simulink model "wModel_C510_BusinesJetw"  (R2020b)
settings: Solver=ode4  StartTime=0.0  StopTime=Tsim  FixedStep=0.005  RelTol=1e-3
values from neighbouring files (symbols this model uses):
  EnginePosition_Left = [-2.2; -1.26; -1.18*0]    [Model_Init00.m]
  EnginePosition_Right = [-2.2;  1.26; -1.18*0]    [Model_Init00.m]
  lat0 = 52.8259    [Model_Init00.m]
  lon0 = -1.3308    [Model_Init00.m]
  MAC = 1.57    [Model_Init00.m]
  MassKg = 3000    [Model_Init00.m]
  WingArea = 19.50    (= 19.5)    [Model_Init00.m]
  WingSpan = 13.20    (= 13.2)    [Model_Init00.m]
undefined symbols (not defined in the file or in its folder): Dx_cg, Earth, trim, WGS84
libraries: aerolibasang x3, aerolibfltsims x2, shared6dof x1, aerolibtransform2 x1, aerolibatmos2 x1
settings Model: Creator=nabram00  LastModifiedBy=kknos
settings DebuggingCC: ArithmeticOperatorsInVariantConditions=warning
settings SFSimCC: CustomCodeUndefinedFunction=UseInterfaceOnly

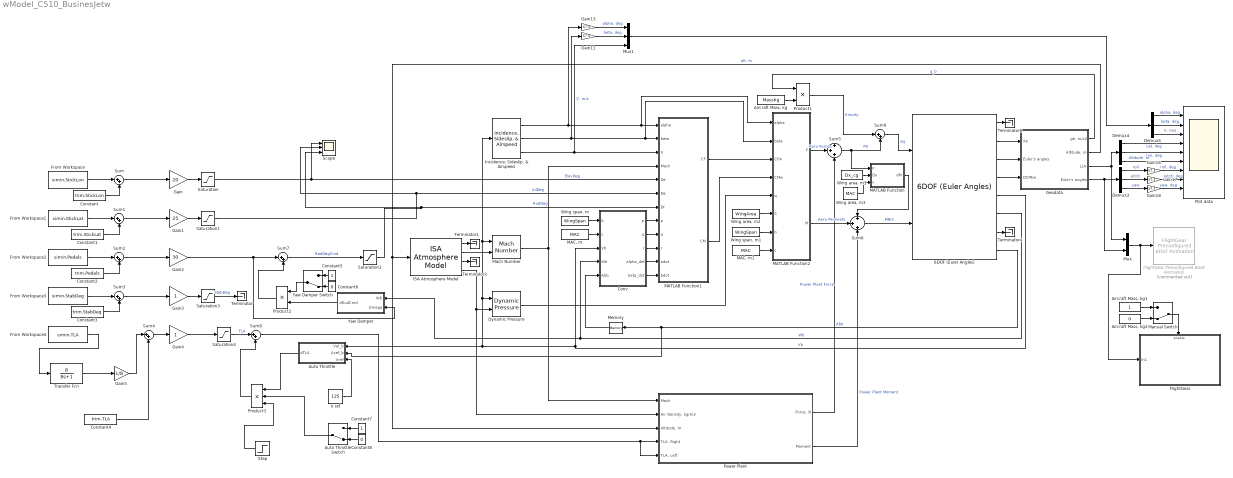
== system wModel_C510_BusinesJetw ==
  " Yaw Damper Switch" : ManualSwitch  CurrentSetting=0
  6DOF (Euler Angles) : shared6dof/6DOF (Euler Angles)  units=Metric (MKS)  mtype=Fixed  rep=Euler Angles  xme_0=trim.PositionE  Vm_0=trim.Vb  eul_0=trim.AttitudeBE  pm_0=trim.OmegaB  mass_0=MassKg  mass_e=0.5  mass_f=2.0  inertia=MoIKgM2  inertia_e=eye(3)  inertia_f=2*eye(3)  k_quat=1.0  vre_flag=on  abi_flag=off  aMode=0  xme_statename=''  Vm_statename=''  eul_statename=''  quat_statename=''  pm_statename=''  mass_statename=''
      settings: SourceProductBaseCode=AE,PW,MT,UV,VE,VP
  "Aircraft Mass, kg" : Constant  Value=MassKg
  "Aircraft Mass, kg1" : Constant  OutDataTypeStr=boolean
  "Aircraft Mass, kg2" : Constant  Value=0  OutDataTypeStr=boolean
  Auto Throttle : Subsystem
  Auto Throttle Switch : ManualSwitch  CurrentSetting=0
  Constant : Constant  Value=trim.StickLon
  Constant1 : Constant  Value=trim.StickLat
  Constant2 : Constant  Value=trim.Pedals
  Constant3 : Constant  Value=trim.StabDeg
  Constant4 : Constant  Value=trim.TLA
  Constant5 : Constant
  Constant6 : Constant  Value=0
  Constant7 : Constant
  Constant8 : Constant  Value=0
  Conv : MATLAB Function  TreatAsAtomicUnit=on
  Demux3 : Demux  Outputs=3
  Demux4 : Demux  Outputs=3
  Demux5 : Demux  Outputs=3
  Dynamic Pressure : aerolibasang/Dynamic Pressure
  FlightGear : Subsystem  TreatAsAtomicUnit=on
  FlightGear Preconfigured 6DoF Animation : aerolibfltsims/FlightGear Preconfigured 6DoF Animation  Commented=on  xFlightGearVersion=v2018.1  DestinationIpAddress=127.0.0.1  DestinationPort=5502  SampleTime=1/25  packetVersion=24
  From Workspace : FromWorkspace  VariableName=simin.StickLon
  From Workspace1 : FromWorkspace  VariableName=simin.StickLat
  From Workspace2 : FromWorkspace  VariableName=simin.Pedals
  From Workspace3 : FromWorkspace  VariableName=simin.StabDeg
  From Workspace4 : FromWorkspace  VariableName=simin.TLA
  Gain : Gain  Gain=20
  Gain1 : Gain  Gain=25
  Gain{11,13,16..18} (5 alike) : Gain  Gain=57.3
  Gain2 : Gain  Gain=30
  Gain3 : Gain
  Gain4 : Gain
  Gain5 : Gain  Gain=1/8
  Geodata : Subsystem  TreatAsAtomicUnit=on
  ISA Atmosphere Model : aerolibatmos2/ISA Atmosphere Model  custom=off  g=9.80665  gamma=1.4  R=287.0531  L=0.0065  h_trop=11000  h_strat=20000  rho0=1.225  P0=101325  T0=288.15  h0=0
  "Incidence, Sideslip, & Airspeed" : aerolibasang/Incidence, Sideslip, & Airspeed
  "MAC, m" : Constant  Value=MAC
  "MAC, m1" : Constant  Value=MAC
  MATLAB Function : MATLAB Function  TreatAsAtomicUnit=on
  MATLAB Function1 : MATLAB Function  TreatAsAtomicUnit=on
  MATLAB Function2 : MATLAB Function  TreatAsAtomicUnit=on
  Mach Number : aerolibasang/Mach Number
      settings: SourceProductBaseCode=AE
  Manual Switch : ManualSwitch  CurrentSetting=0
  Memory : Memory
  Mux : Mux  Inputs=2
  Mux1 : Mux  Inputs=3
  Plot data : Scope  NumInputPorts=9
  Power Plant : Subsystem  TreatAsAtomicUnit=on
  Product1 : Product
  Product2 : Product
  Product3 : Product  Inputs=3
  Saturation : Saturate  UpperLimit=20  LowerLimit=-20
  Saturation1 : Saturate  UpperLimit=25  LowerLimit=-25
  Saturation2 : Saturate  UpperLimit=30  LowerLimit=-30
  Saturation3 : Saturate  UpperLimit=3  LowerLimit=-8
  Saturation4 : Saturate  UpperLimit=1  LowerLimit=0
  Scope : Scope  NumInputPorts=3
  Step : Step  Time=0.1  SampleTime=0
  Sum{,1..4,7..9} (8 alike) : Sum  Inputs=|++
  Sum5 : Sum  Inputs=+|+|+
  Sum6 : Sum  Inputs=+|+|+
  Terminator{,1,3..4,6} (5 alike) : Terminator
  Transfer Fcn : TransferFcn  Numerator=[8]  Denominator=[8 1]
  V ref : Constant  Value=125
  "Wing area, m1" : Constant  Value=Dx_cg
  "Wing area, m2" : Constant  Value=WingArea
  "Wing area, m3" : Constant  Value=MAC
  "Wing span, m" : Constant  Value=WingSpan
  "Wing span, m1" : Constant  Value=WingSpan
  Yaw Damper : Subsystem
  wires:
  From Workspace/1 -> Sum/1
  From Workspace1/1 -> Sum1/1
  From Workspace2/1 -> Sum2/1
  From Workspace3/1 -> Sum3/1
  Constant/1 -> Sum/2
  Constant1/1 -> Sum1/2
  Constant2/1 -> Sum2/2
  Constant3/1 -> Sum3/2
  Constant4/1 -> Sum4/2
  Sum/1 -> Gain/1
  Sum1/1 -> Gain1/1
  Sum2/1 -> Gain2/1
  Sum3/1 -> Gain3/1
  Sum4/1 -> Gain4/1
  Gain/1 -> Saturation/1
  Gain1/1 -> Saturation1/1
  Gain3/1 -> Saturation3/1
  Gain4/1 -> Saturation4/1
  Saturation/1 -> MATLAB Function1/5(De), Scope/1  "ElevDeg"
  Saturation1/1 -> Scope/2, MATLAB Function1/6(Da)  "AilDeg"
  Saturation2/1 -> Scope/3, MATLAB Function1/7(Dr)  "RudDeg"
  Saturation3/1 -> Terminator/1  "StabDeg"
  ISA Atmosphere Model/4 -> Power Plant/2("Air Density, kg/m3"), Dynamic Pressure/2
  ISA Atmosphere Model/3 -> Terminator3/1
  ISA Atmosphere Model/2 -> Mach Number/2
  ISA Atmosphere Model/1 -> Terminator1/1
  Geodata/2("Altitude, m") -> ISA Atmosphere Model/1, Power Plant/3("Altitude, m")  "alt, m"
  MATLAB Function1/1(CF) -> MATLAB Function2/3(CFw)
  MATLAB Function1/2(CM) -> MATLAB Function2/4(CMw)
  Sum6/1 -> 6DOF (Euler Angles)/2  "MNm"
  6DOF (Euler Angles)/6 -> Conv/4(Wb), Yaw Damper/1(Wb)  "Wb"
  Conv/1(p) -> MATLAB Function1/8(p)
  Conv/2(q) -> MATLAB Function1/9(q)
  Conv/3(r) -> MATLAB Function1/10(r)
  Mach Number/1 -> MATLAB Function1/4(Mach), Power Plant/1(Mach)
  Dynamic Pressure/1 -> MATLAB Function2/5(q)
  6DOF (Euler Angles)/5 -> Auto Throttle/1(Vel_b), Mach Number/1, "Incidence, Sideslip, & Airspeed"/1, Dynamic Pressure/1, Conv/3(Vb)  "Vb"
  "Incidence, Sideslip, & Airspeed"/1 -> MATLAB Function1/1(alpha), MATLAB Function2/1(alpha), Gain13/1
  "Incidence, Sideslip, & Airspeed"/2 -> MATLAB Function1/2(beta), MATLAB Function2/2(beta), Gain11/1
  "Incidence, Sideslip, & Airspeed"/3 -> Mux1/3, MATLAB Function1/3(V)  "V, m/s"
  Mux/1 -> FlightGear/1(In1), FlightGear Preconfigured 6DoF Animation/1
  Conv/4(alpha_dot) -> MATLAB Function1/11(adot)
  Conv/5(beta_dot) -> MATLAB Function1/12(bdot)
  "Wing span, m1"/1 -> MATLAB Function2/7(b)
  "MAC, m1"/1 -> MATLAB Function2/8(c)
  Gain13/1 -> Mux1/1  "alpha, deg"
  MATLAB Function2/2(M) -> Sum6/2  "Aero Moments"
  MATLAB Function2/1(F) -> Sum5/2  "Aero Forces"
  6DOF (Euler Angles)/8 -> Auto Throttle/2(Acef_b), Memory/1  "Abb"
  6DOF (Euler Angles)/7 -> Terminator4/1
  6DOF (Euler Angles)/1 -> Terminator6/1
  6DOF (Euler Angles)/3 -> Geodata/2(Euler's angles)
  "Aircraft Mass, kg"/1 -> Product1/2
  Product1/1 -> Sum9/1  "Gravity"
  Demux3/1 -> Gain16/1  "roll"
  Demux3/2 -> Gain17/1  "pitch"
  Demux3/3 -> Gain18/1  "yaw"
  Gain16/1 -> Plot data/7  "roll, deg"
  Gain17/1 -> Plot data/8  "pitch, deg"
  Gain18/1 -> Plot data/9  "yaw, deg"
  Geodata/1("gb, m/s2") -> Product1/1  "g_b"
  6DOF (Euler Angles)/2 -> Geodata/1(Xe)
  6DOF (Euler Angles)/4 -> Geodata/3(DCMbe)
  Geodata/4(Euler's angles) -> Demux3/1, Mux/2
  Geodata/3(LLA) -> Demux4/1, Mux/1
  Demux4/1 -> Plot data/4  "Lat, deg"
  Demux4/2 -> Plot data/5  "Lon, deg"
  Demux4/3 -> Plot data/6  "Altitude, m"
  "Wing span, m"/1 -> Conv/1(b)
  "Wing area, m2"/1 -> MATLAB Function2/6(S)
  "MAC, m"/1 -> Conv/2(c)
  Power Plant/1("Force, N") -> Sum5/3  "Power Plant Force"
  Power Plant/2(Moment) -> Sum6/3  "Power Plant Moment"
  Mux1/1 -> Demux5/1
  Demux5/3 -> Plot data/3  "V, m/s"
  Demux5/2 -> Plot data/2  "beta, deg"
  Demux5/1 -> Plot data/1  "alpha, deg"
  Gain11/1 -> Mux1/2  "beta, deg"
  Manual Switch/1 -> FlightGear/Enable
  "Aircraft Mass, kg2"/1 -> Manual Switch/2
  "Aircraft Mass, kg1"/1 -> Manual Switch/1
  Memory/1 -> Conv/5(Abb)
  Gain2/1 -> Sum7/1, Yaw Damper/2(Omega)
  Sum7/1 -> Saturation2/1  "RadDegCmd"
  Yaw Damper/1(dRudCmd) -> Product2/2
  Constant5/1 -> " Yaw Damper Switch"/1
  Constant6/1 -> " Yaw Damper Switch"/2
  " Yaw Damper Switch"/1 -> Product2/1
  Product2/1 -> Sum7/2
  Constant8/1 -> Auto Throttle Switch/2
  Constant7/1 -> Auto Throttle Switch/1
  Auto Throttle/1(dTLA) -> Product3/1
  Product3/1 -> Sum8/2
  Saturation4/1 -> Sum8/1  "TLA"
  V ref/1 -> Auto Throttle/3(Vref)
  Transfer Fcn/1 -> Gain5/1
  Sum9/1 -> 6DOF (Euler Angles)/1  "FN"
  Sum5/1 -> MATLAB Function/1(F), Sum9/2  "FN"
  "Wing area, m1"/1 -> MATLAB Function/2(Dx)
  "Wing area, m3"/1 -> MATLAB Function/3(c)
  MATLAB Function/1(dM) -> Sum6/1
  From Workspace4/1 -> Transfer Fcn/1
  Auto Throttle Switch/1 -> Product3/2
  Gain5/1 -> Sum4/1
  Sum8/1 -> Power Plant/5("TLA, Left"), Power Plant/4("TLA, Right")
  Step/1 -> Product3/3

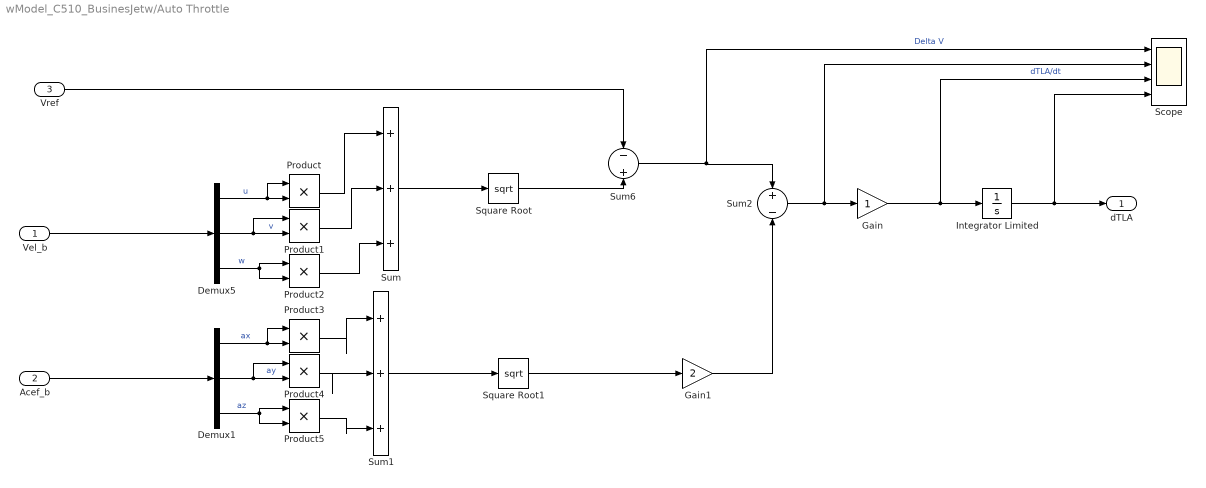
== system wModel_C510_BusinesJetw/Auto Throttle ==
  Vel_b : Inport
  Acef_b : Inport  Port=2
  Vref : Inport  Port=3
  Demux1 : Demux  Outputs=3
  Demux5 : Demux  Outputs=3
  Gain : Gain
  Gain1 : Gain  Gain=2
  Integrator Limited : Integrator  LimitOutput=on  UpperSaturationLimit=1  LowerSaturationLimit=0
  Product{,1..5} (6 alike) : Product
  Scope : Scope  NumInputPorts=4
  Square Root : Sqrt  SaturateOnIntegerOverflow=on
  Square Root1 : Sqrt  SaturateOnIntegerOverflow=on
  Sum : Sum  Inputs=|+++
  Sum1 : Sum  Inputs=|+++
  Sum2 : Sum  Inputs=+|-
  Sum6 : Sum  Inputs=-|+
  dTLA : Outport
  wires:
  Demux5/3 -> Product2/1, Product2/2  "w"
  Demux5/1 -> Product/1, Product/2  "u"
  Demux5/2 -> Product1/1, Product1/2  "v"
  Demux1/1 -> Product3/1, Product3/2  "ax"
  Demux1/3 -> Product5/1, Product5/2  "az"
  Demux1/2 -> Product4/1, Product4/2  "ay"
  Product1/1 -> Sum/2
  Product/1 -> Sum/1
  Product2/1 -> Sum/3
  Product3/1 -> Sum1/1
  Product4/1 -> Sum1/2
  Product5/1 -> Sum1/3
  Sum/1 -> Square Root/1
  Sum1/1 -> Square Root1/1
  Vref/1 -> Sum6/1
  Square Root/1 -> Sum6/2
  Sum6/1 -> Sum2/1, Scope/1  "Delta V"
  Square Root1/1 -> Gain1/1
  Gain1/1 -> Sum2/2
  Sum2/1 -> Scope/2, Gain/1
  Gain/1 -> Integrator Limited/1, Scope/3  "dTLA/dt"
  Vel_b/1 -> Demux5/1
  Acef_b/1 -> Demux1/1
  Integrator Limited/1 -> Scope/4, dTLA/1

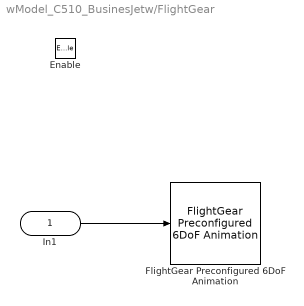
== system wModel_C510_BusinesJetw/FlightGear ==
  In1 : Inport
  Enable : EnablePort
  FlightGear Preconfigured 6DoF Animation : aerolibfltsims/FlightGear Preconfigured 6DoF Animation  xFlightGearVersion=v2018.1  DestinationIpAddress=127.0.0.1  DestinationPort=5502  SampleTime=1/25  packetVersion=24
  wires:
  In1/1 -> FlightGear Preconfigured 6DoF Animation/1

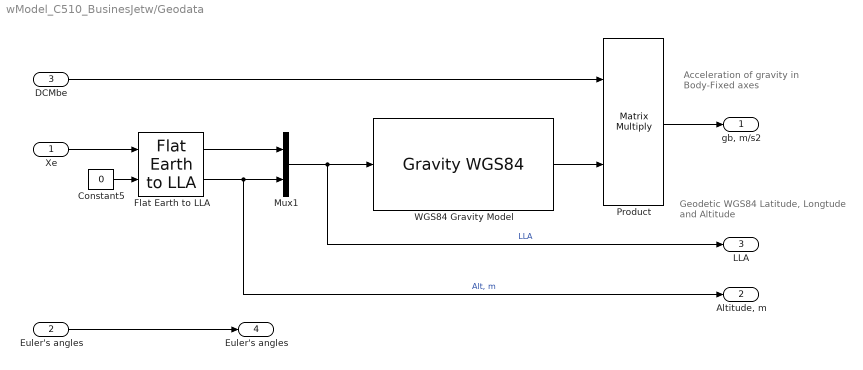
== system wModel_C510_BusinesJetw/Geodata ==
  note: Geodetic WGS84
      | Latitude, Longtude and Altitude
  note: Acceleration of gravity
      | in Body-Fixed axes
  Xe : Inport
  Euler's angles : Inport  Port=2
  DCMbe : Inport  Port=3
  Constant5 : Constant  Value=0
  Flat Earth to LLA : aerolibtransform2/Flat Earth to LLA  units=Metric (MKS)  ptype=Earth (WGS84)  F=1/298.257223563  R=6378137  refPosPort=off  LL0=[lat0 lon0]  psi=0
  Mux1 : Mux  Inputs=2
  Product : Product  Multiplication=Matrix(*)
  "WGS84 Gravity Model  " : GravityWGS84
  "gb, m/s2" : Outport  VectorParamsAs1DForOutWhenUnconnected=off
  "Altitude, m" : Outport  Port=2  VectorParamsAs1DForOutWhenUnconnected=off
  LLA : Outport  Port=3  VectorParamsAs1DForOutWhenUnconnected=off
  Euler's angles : Outport  Port=4  VectorParamsAs1DForOutWhenUnconnected=off
  wires:
  Xe/1 -> Flat Earth to LLA/1
  DCMbe/1 -> Product/1
  Product/1 -> "gb, m/s2"/1
  Flat Earth to LLA/1 -> Mux1/1
  Constant5/1 -> Flat Earth to LLA/2
  "WGS84 Gravity Model  "/1 -> Product/2
  Flat Earth to LLA/2 -> Mux1/2, "Altitude, m"/1  "Alt, m"
  Mux1/1 -> "WGS84 Gravity Model  "/1, LLA/1  "LLA"
  Euler's angles/1 -> Euler's angles/1

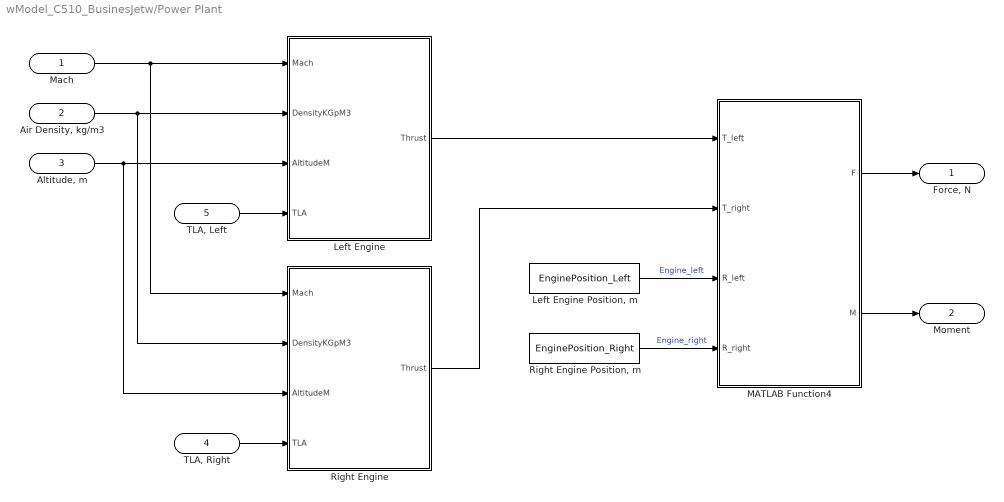
== system wModel_C510_BusinesJetw/Power Plant ==
  Mach : Inport
  "Air Density, kg/m3" : Inport  Port=2
  "Altitude, m" : Inport  Port=3
  "TLA, Right" : Inport  Port=4
  "TLA, Left" : Inport  Port=5
  Left Engine : MATLAB Function  TreatAsAtomicUnit=on
  "Left Engine Position, m" : Constant  Value=EnginePosition_Left
  MATLAB Function4 : MATLAB Function  TreatAsAtomicUnit=on
  Right Engine : MATLAB Function  TreatAsAtomicUnit=on
  "Right Engine Position, m" : Constant  Value=EnginePosition_Right
  "Force, N" : Outport  VectorParamsAs1DForOutWhenUnconnected=off
  Moment : Outport  Port=2  VectorParamsAs1DForOutWhenUnconnected=off
  wires:
  "Left Engine Position, m"/1 -> MATLAB Function4/3(R_left)  "Engine_left"
  "Right Engine Position, m"/1 -> MATLAB Function4/4(R_right)  "Engine_right"
  MATLAB Function4/1(F) -> "Force, N"/1
  Mach/1 -> Left Engine/1(Mach), Right Engine/1(Mach)
  "Air Density, kg/m3"/1 -> Left Engine/2(DensityKGpM3), Right Engine/2(DensityKGpM3)
  "Altitude, m"/1 -> Left Engine/3(AltitudeM), Right Engine/3(AltitudeM)
  "TLA, Left"/1 -> Left Engine/4(TLA)
  "TLA, Right"/1 -> Right Engine/4(TLA)
  MATLAB Function4/2(M) -> Moment/1
  Left Engine/1(Thrust) -> MATLAB Function4/1(T_left)
  Right Engine/1(Thrust) -> MATLAB Function4/2(T_right)

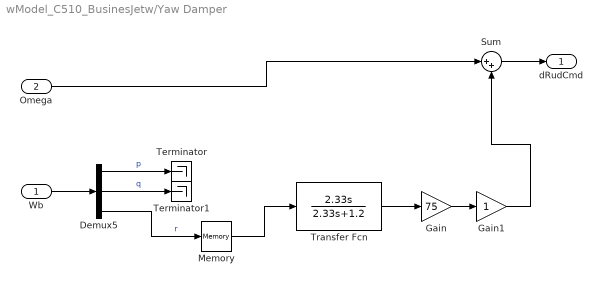
== system wModel_C510_BusinesJetw/Yaw Damper ==
  Wb : Inport
  Omega : Inport  Port=2
  Demux5 : Demux  Outputs=3
  Gain : Gain  Gain=75
  Gain1 : Gain
  Memory : Memory
  Sum : Sum  Inputs=|++
  Terminator : Terminator
  Terminator1 : Terminator
  Transfer Fcn : TransferFcn  Numerator=[2.33 0]  Denominator=[2.33 1.2]
  dRudCmd : Outport
  wires:
  Demux5/1 -> Terminator/1  "p"
  Demux5/3 -> Memory/1  "r"
  Demux5/2 -> Terminator1/1  "q"
  Wb/1 -> Demux5/1
  Transfer Fcn/1 -> Gain/1
  Gain/1 -> Gain1/1
  Gain1/1 -> Sum/2
  Omega/1 -> Sum/1
  Sum/1 -> dRudCmd/1
  Memory/1 -> Transfer Fcn/1

== matlab function wModel_C510_BusinesJetw/MATLAB Function ==
  data: F input; dM output; Dx input; c input
function dM = cg_shift(F,Dx,c)

dM = zeros(3,1);
dM = cross([-Dx*c; 0; 0],F(:));


end

== matlab function wModel_C510_BusinesJetw/MATLAB Function1 ==
  data: alpha input; beta input; V input; CF output; Mach input; De input; CM output; Da input; Dr input; p input; q input; r input; adot input; bdot input
function [CF, CM] = C510aero(alpha, beta, V, Mach, De,Da,Dr, p,q,r, adot,bdot)
%% inputs:
%  alpha, beta  - rad
%  Mach         - undim
%  De,Da,Dr     - deg
%  p,q,r        - undim
%  adot         - undim
%  bdot         - undim


AlphaTable = [-10    -8    -6    -4    -2     0     2     4     6     8    10    11    12    13    14    15    16    17    18    19    20    21    22    23    24    25    30    35    40    45    50    55    60    65    70    75    80    85    90];

%% Drag force
% Drag_at_zero_lift
CD0 = 0;

% Drag_due_to_alpha
CDTable = [ 0.0814    0.0613    0.0458    0.0347    0.0280    0.0258    0.0280    0.0347    0.0458    0.0613    0.0705    0.0811    0.0933    0.1073    0.1180    0.1298    0.1428    0.1571    0.1728    0.1901    0.2091    0.2300    0.2530    0.2783  0.3061    0.3392    0.5617    0.8479    1.1934    1.5886    2.0199    2.4698    2.9185    3.3450    3.7284    4.0495    4.2916    4.4422    4.4933];
CDwbh = interp1(AlphaTable, CDTable, rad2deg(alpha));

% Drag_due_to_Elevator_Deflection, per rad
CDDe = 0.07;

% Drag_due_to_sideslip
CDbeta = 0.16;

CD = CD0 + CDwbh + CDDe*deg2rad(De) + CDbeta*abs(beta);



%% Side force
% Side_force_due_to_beta
CYBetaTable = [-0.6489   -0.6525   -0.6553   -0.6573   -0.6585   -0.6589   -0.6585   -0.6573   -0.6553   -0.6525   -0.6489   -0.6468   -0.6445   -0.6420   -0.6393   -0.6364   -0.6334   -0.6301   -0.6266   -0.6230   -0.6191   -0.6151   -0.6109   -0.6065 -0.6019   -0.5971   -0.5706   -0.5397   -0.5047   -0.4659   -0.4235   -0.3779   -0.3294   -0.2785   -0.2254   -0.1705   -0.1144   -0.0574    0.0000];
CYb = interp1(AlphaTable, CYBetaTable, rad2deg(alpha));

% Side_force_due_to_aileron
CYda = -0.043;

% Side_force_due_to_rudder
CYdr = 0.1574;

% Side_force_due_to_roll_rate
CYp = -0.04;

% Side_force_due_to_yaw_rate
CYr = 0.233;

CY = CYb*beta + CYda*deg2rad(Da) + CYdr*deg2rad(Dr) + CYp*p + CYr*r;



%% Lift(alpha, De, adot, q)
% Lift_due_to_alpha
CLTable = [-1.1041   -0.8833   -0.6625   -0.4417   -0.2208   0    0.2208    0.4417    0.6625    0.8833    1.1041    1.2117    1.2885    1.3346    1.3500    1.3346    1.2885    1.2117    1.1041    0.9659    0.7968    0.7300    0.7300    0.7400    0.7600    0.7800    0.9728    1.2109    1.4222    1.5886    1.6949    1.7294    1.6850    1.5598    1.3570    1.0850    0.7567    0.3886   -0.0000];
CLwbh = interp1(AlphaTable, CLTable, rad2deg(alpha));

% Lift_due_to_Elevator_Deflection
CLDeTable = [0.4885    0.4912    0.4933    0.4948    0.4957    0.4956    0.4951    0.4937    0.4915    0.4882    0.4835    0.4805    0.4769    0.4727    0.4677    0.4619    0.4550    0.4468    0.4373    0.4263    0.4136    0.3994    0.3837    0.3667    0.3488    0.3306    0.2505    0.2058    0.1827    0.1660    0.1503    0.1339    0.1167    0.0987    0.0798    0.0604    0.0405    0.0203   -0.0000];
CLDe = interp1(AlphaTable, CLDeTable, rad2deg(alpha));

% Lift_due_to_alpha_rate
CLadot = 2.24;

% Lift_due_to_pitch_rate
CLq  = 4.49;

CL = CLwbh + CLDe*deg2rad(De) + CLadot*adot + CLq*q;



%% Roll
% Roll_moment_due_to_beta
ClBetaTable = [0.0027   -0.0068   -0.0164   -0.0261   -0.0358   -0.0454   -0.0550   -0.0646   -0.0740   -0.0832   -0.0922   -0.0965   -0.0995   -0.1011   -0.1013   -0.1002   -0.0978   -0.0940   -0.0891   -0.0828   -0.0754   -0.0722   -0.0717   -0.0716  -0.0718   -0.0720   -0.0761   -0.0805   -0.0824   -0.0812   -0.0768   -0.0694   -0.0595   -0.0480   -0.0358   -0.0240   -0.0136   -0.0054    0.0000];
Clb = interp1(AlphaTable, ClBetaTable, rad2deg(alpha));

% Roll_moment_due_to_roll_rate_(roll_damping)
ClpTable = [-0.7476   -0.7517   -0.7549   -0.7572   -0.7586   -0.7591   -0.7586   -0.7572   -0.7549   -0.7517   -0.7476   -0.7452   -0.7425   -0.7396   -0.7365   -0.7332   -0.7297   -0.7259   -0.7219   -0.7177   -0.7133   -0.7087   -0.7038   -0.6988    -0.6935   -0.6880   -0.6574   -0.6218   -0.5815   -0.5368   -0.4879   -0.4354   -0.3795   -0.3208   -0.2596   -0.1965   -0.1318   -0.0662    0.0000];
Clp = interp1(AlphaTable, ClpTable, rad2deg(alpha));

% Roll_moment_due_to_yaw_rate
ClrTable = [-0.7476   -0.7517   -0.7549   -0.7572   -0.7586   -0.7591   -0.7586   -0.7572   -0.7549   -0.7517   -0.7476   -0.7452   -0.7425   -0.7396   -0.7365   -0.7332   -0.7297   -0.7259   -0.7219   -0.7177   -0.7133   -0.7087   -0.7038   -0.6988    -0.6935   -0.6880   -0.6574   -0.6218   -0.5815   -0.5368   -0.4879   -0.4354   -0.3795   -0.3208   -0.2596   -0.1965   -0.1318   -0.0662    0.0000];
Clr = interp1(AlphaTable, ClrTable, rad2deg(alpha));

% Roll_moment_due_to_aileron
ClDaTable = [0.1099    0.1105    0.1110    0.1113    0.1115    0.1116    0.1115    0.1113    0.1110    0.1105    0.1099    0.1095    0.1091    0.1087    0.1083    0.1078    0.1073    0.1067    0.1061    0.1055    0.1048    0.1042    0.1035    0.1027    0.1019    0.1011    0.0966    0.0914    0.0855    0.0789    0.0717    0.0640    0.0558    0.0472    0.0382    0.0289    0.0194    0.0097   -0.0000];
Clda = interp1(AlphaTable, ClDaTable, rad2deg(alpha));

% Roll_moment_due_to_rudder
ClDrTable = [-0.0383   -0.0385   -0.0386   -0.0388   -0.0388   -0.0389   -0.0388   -0.0388   -0.0386   -0.0385   -0.0383   -0.0381   -0.0380   -0.0379   -0.0377   -0.0375   -0.0374   -0.0372   -0.0370   -0.0367   -0.0365   -0.0363   -0.0360   -0.0358    -0.0355   -0.0352   -0.0337   -0.0318   -0.0298   -0.0275   -0.0250   -0.0223   -0.0194   -0.0164   -0.0133   -0.0101   -0.0067   -0.0034    0.0000];
Cldr = interp1(AlphaTable, ClDrTable, rad2deg(alpha));

Cl = Clb*beta + Clda*deg2rad(Da) + Cldr*deg2rad(Dr) + Clp*p + Clr*r;



%% Pitch moment (alpha, q, adot, De)
% Pitching_moment_at_zero_alpha
Cmo = 0.02;

% Pitch_moment_due_to_alpha
CmTable = [0.1467    0.1176    0.0884    0.0590    0.0295         0   -0.0295   -0.0590   -0.0884   -0.1176   -0.1464   -0.1605   -0.1704   -0.1764   -0.1782   -0.1761   -0.1702   -0.1604   -0.1469   -0.1299   -0.1092   -0.0983   -0.0885   -0.0796          -0.0717   -0.0755   -0.1223   -0.1940   -0.2537   -0.3070   -0.3603   -0.4120   -0.4605   -0.5043   -0.5421   -0.5728   -0.5954   -0.6093   -0.6139];
Cmalpha = interp1(AlphaTable, CmTable, rad2deg(alpha));

% Pitch_moment_due_to_pitch_rate
Cmq = -13.17;

% Pitch_moment_due_to_alpha_rate
Cmadot = -7.42;

% Pitch_moment_due_to_elevator_deflection
CmDeTable = [-1.5323   -1.5408   -1.5474   -1.5521   -1.5549   -1.5547   -1.5530   -1.5488   -1.5417   -1.5313   -1.5166   -1.5071   -1.4960   -1.4828   -1.4672   -1.4488   -1.4271   -1.4015   -1.3717   -1.3371   -1.2975   -1.2528   -1.2034   -1.1501   -1.0941   -1.0369   -0.7858   -0.6456   -0.5731   -0.5208   -0.4714   -0.4201   -0.3661   -0.3094   -0.2504   -0.1895   -0.1271   -0.0638    0.0000];
Cmde = interp1(AlphaTable, CmDeTable, rad2deg(alpha));

Cm = Cmo + Cmalpha + Cmq*q + Cmadot*adot + Cmde*deg2rad(De);



%% Yaw moment
% Yaw_moment_due_to_beta
CnBetaTable = [0.0945    0.0959    0.0972    0.0983    0.0994    0.1003    0.1011    0.1018    0.1023    0.1028    0.1030    0.1031    0.1031    0.1028    0.1025    0.1019    0.1013    0.1005    0.0995    0.0984    0.0972    0.0963    0.0957    0.0950    0.0944    0.0937    0.0902    0.0861    0.0811    0.0753    0.0687    0.0614    0.0535    0.0450    0.0361    0.0271    0.0179    0.0089   -0.0000];
Cnb = interp1(AlphaTable, CnBetaTable, rad2deg(alpha));

% Yaw_moment_due_to_roll_rate
CnpTable = [0.1536    0.1236    0.0931    0.0623    0.0312         0   -0.0312   -0.0623   -0.0931   -0.1236   -0.1536   -0.1681   -0.1781   -0.1838   -0.1851   -0.1822   -0.1750   -0.1637   -0.1484   -0.1290   -0.1058   -0.0963   -0.0956   -0.0963   -0.0981   -0.0999   -0.1190   -0.1402   -0.1539   -0.1587   -0.1539   -0.1402   -0.1190   -0.0931   -0.0656   -0.0397   -0.0186   -0.0048   -0.0000];
Cnp = interp1(AlphaTable, CnpTable, rad2deg(alpha));

% Yaw_moment_due_to_yaw_rate
CnrTable = [-0.1883   -0.1445   -0.1102   -0.0855   -0.0706   -0.0656   -0.0706   -0.0855   -0.1102   -0.1445   -0.1883   -0.2128   -0.2314   -0.2427   -0.2458   -0.2406   -0.2274   -0.2074   -0.1818   -0.1529   -0.1231   -0.1125   -0.1117   -0.1123    -0.1143   -0.1162   -0.1412   -0.1775   -0.2098   -0.2302   -0.2324   -0.2143   -0.1790   -0.1336   -0.0873   -0.0484   -0.0216   -0.0071    0.0000];
Cnr = interp1(AlphaTable, CnrTable, rad2deg(alpha));

% Yaw_moment_due_to_aileron
CnDaTable   = [0     0     0     0     0     0     0     0     0     0     0     0     0     0     0     0     0     0     0     0     0     0     0     0     0     0     0     0     0     0     0     0     0     0     0     0     0     0     0];
Cnda = interp1(AlphaTable, CnDaTable, rad2deg(alpha));

% Yaw_moment_due_to_rudder
CnDrTable   = [-0.0917   -0.0922   -0.0926   -0.0929   -0.0931   -0.0931   -0.0931   -0.0929   -0.0926   -0.0922   -0.0917   -0.0914   -0.0911   -0.0907   -0.0904   -0.0900   -0.0895   -0.0891   -0.0886   -0.0881   -0.0875   -0.0869   -0.0863   -0.0857    -0.0851   -0.0844   -0.0807   -0.0763   -0.0713   -0.0659   -0.0599   -0.0534   -0.0466   -0.0394   -0.0319   -0.0241   -0.0162   -0.0081    0.0000];
Cndr = interp1(AlphaTable, CnDrTable, rad2deg(alpha));

Cn  = Cnb*beta + Cnp*p + Cnr*r + Cnda*deg2rad(Da) + Cndr*deg2rad(Dr);



%% In wind axes
CF = [CD CY CL]';
CM = [Cl Cm Cn]';

end

== matlab function wModel_C510_BusinesJetw/Power Plant/Left Engine ==
  data: Mach input; DensityKGpM3 input; AltitudeM input; TLA input; Thrust output
function Thrust  = BJprop(Mach,DensityKGpM3,AltitudeM,TLA)

StaticThrust = 6490;	% Static thrust at sea level, N	
Thrust       = TLA*StaticThrust*(DensityKGpM3/1.225)^0.7*(1-exp((AltitudeM-17000)/2000)); 	% Thrust at Altitude, N 

end

== matlab function wModel_C510_BusinesJetw/MATLAB Function2 ==
  data: alpha input; beta input; CFw input; F output; CMw input; q input; S input; b input; c input; M output
function [F,M] = Conv2Dim(alpha, beta, CFw, CMw, q, S, b, c)
% Computation of dimensional forces and moments

F = zeros(3,1);
M = zeros(3,1);

% Convertion from wind to body frame, ignore sideslip
CX = -CFw(1)*cos(alpha) + CFw(3)*sin(alpha);
CY =  CFw(2);
CZ = -CFw(1)*sin(alpha) - CFw(3)*cos(alpha);

% Dimensional aerodynamic forces and moments
F(1) = CX * q*S;  % N
F(2) = CY * q*S;  % N
F(3) = CZ * q*S;  % N

M(1) = CMw(1) * q*S*b;  % Nm
M(2) = CMw(2) * q*S*c;  % Nm
M(3) = CMw(3) * q*S*b;  % Nm
 
end

== matlab function wModel_C510_BusinesJetw/Power Plant/Right Engine ==
  data: Mach input; DensityKGpM3 input; AltitudeM input; TLA input; Thrust output
function Thrust  = BJprop(Mach,DensityKGpM3,AltitudeM,TLA)

StaticThrust = 6490;	% Static thrust at sea level, N	
Thrust       = TLA*StaticThrust*(DensityKGpM3/1.225)^0.7*(1-exp((AltitudeM-17000)/2000)); 	% Thrust at Altitude, N 

end

== matlab function wModel_C510_BusinesJetw/Power Plant/MATLAB Function4 ==
  data: T_left input; T_right input; R_left input; R_right input; F output; M output
function [F,M] = PowerPlantFM(T_left, T_right, R_left, R_right)

F = zeros(3,1);
M = zeros(3,1);

% Total force (Thrust axes is parallel to xb)
F(1) = T_left + T_right; % N

% Moments from left and right engine, Nm
M_left  = cross(R_left,  [T_left;  0; 0]);
M_right = cross(R_right, [T_right; 0; 0]);

% Total moments, Nm
M = M_left + M_right;

end

== matlab function wModel_C510_BusinesJetw/Conv ==
  data: b input; c input; Vb input; p output; q output; r output; Wb input; alpha_dot output; beta_dot output; Abb input
function [p,q,r, alpha_dot, beta_dot] = conv2undim(b,c, Vb,Wb,Abb)

%% Additional states, [u,v,w] - m/s, [u_dot,v_dot,w_dot] - m/s2
u = Vb(1);          u_dot = Abb(1);
v = Vb(2);          v_dot = Abb(2);
w = Vb(3);          w_dot = Abb(3);

V     = sqrt(u^2 + v^2 + w^2);
V_dot = (u*u_dot + v*v_dot + w*w_dot)/V;

% nondimensional
alpha_dot = c/(2*V) * (u*w_dot - w*u_dot)/(u^2+w^2);
beta_dot  = b/(2*V) * (V*v_dot - v*V_dot)/(V*sqrt(u^2+w^2));


%% Convertion of angular rates:
%  Body-fixed Wb = [p,q,r] from rad/s to nondimensional ones
p = Wb(1) * b/(2*V);
q = Wb(2) * c/(2*V);
r = Wb(3) * b/(2*V);

end
